simulink model "physics"  (R2015a)
settings: Solver=ode45  StartTime=0.0  StopTime=10.0  RelTol=1e-3
undefined symbols (not defined in the file or in its folder): Kd, Lyaw
libraries: simulink x2
settings Model: Creator=Cassandra  LastModifiedBy=Cassandra

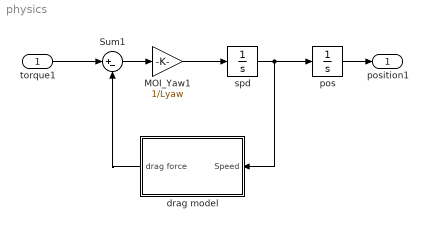
== system physics ==
  torque1 : Inport
  MOI_Yaw1 : Gain  Gain=1/Lyaw
  Sum1 : Sum  Inputs=|+-
  drag model : Subsystem
  pos : Integrator
  spd : Integrator
  position1 : Outport
  wires:
  spd/1 -> pos/1, drag model/1(Speed)
  MOI_Yaw1/1 -> spd/1
  pos/1 -> position1/1
  Sum1/1 -> MOI_Yaw1/1
  drag model/1(drag force) -> Sum1/2
  torque1/1 -> Sum1/1

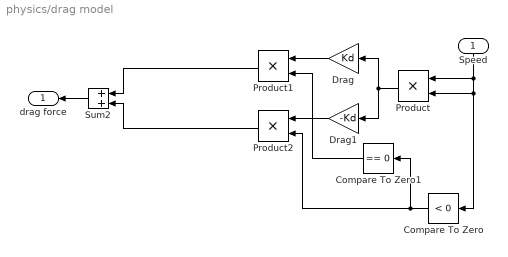
== system physics/drag model ==
  Speed : Inport
  Compare To Zero : simulink/Logic and Bit Operations/Compare To Zero  relop=<  OutDataTypeStr=boolean
  Compare To Zero1 : simulink/Logic and Bit Operations/Compare To Zero  relop===  OutDataTypeStr=boolean
  Drag : Gain  Gain=Kd
  Drag1 : Gain  Gain=-Kd
  Product : Product
  Product1 : Product
  Product2 : Product
  Sum2 : Sum  Inputs=+|+
  drag force : Outport
  wires:
  Speed/1 -> Product/1, Compare To Zero/1, Product/2
  Drag1/1 -> Product2/1
  Compare To Zero1/1 -> Product1/2
  Product1/1 -> Sum2/1
  Drag/1 -> Product1/1
  Sum2/1 -> drag force/1
  Product/1 -> Drag1/1, Drag/1
  Product2/1 -> Sum2/2
  Compare To Zero/1 -> Product2/2, Compare To Zero1/1
